simulink library "INT_ACCmpr_DD"  (R2016b)
settings: Solver=VariableStepAuto  StartTime=0.0  StopTime=10.0  RelTol=1e-3
settings Model: Creator=liutao  LastModifiedBy=liutao

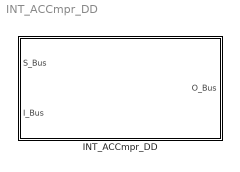
== system INT_ACCmpr_DD ==
  INT_ACCmpr_DD : Subsystem

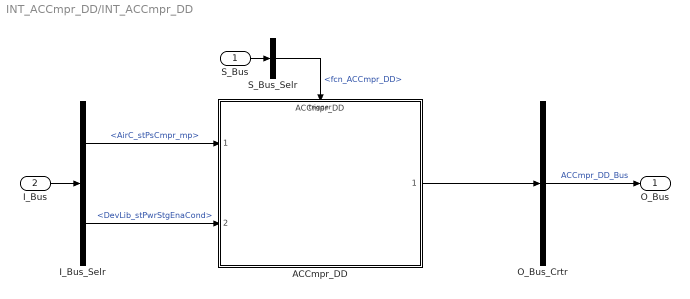
== system INT_ACCmpr_DD/INT_ACCmpr_DD ==
  S_Bus : Inport
  I_Bus : Inport  Port=2
  ACCmpr_DD : ModelReference  ModelNameDialog=ACCmpr_DD  SimulationMode=Normal  ModelReferenceVersion=1.14  TriggerPortName=function  TriggerPortTriggerType=function-call  TriggerPortStatesWhenEnabling=held
  I_Bus_Selr : BusSelector  OutputSignals=AirC_stPsCmpr_mp,DevLib_stPwrStgEnaCond
  O_Bus_Crtr : BusCreator  Inputs=1
  S_Bus_Selr : BusSelector  OutputSignals=fcn_ACCmpr_DD
  O_Bus : Outport
  wires:
  S_Bus_Selr/1 -> ACCmpr_DD/Trigger  "<fcn_ACCmpr_DD>"
  S_Bus/1 -> S_Bus_Selr/1
  I_Bus/1 -> I_Bus_Selr/1
  I_Bus_Selr/1 -> ACCmpr_DD/1  "<AirC_stPsCmpr_mp>"
  I_Bus_Selr/2 -> ACCmpr_DD/2  "<DevLib_stPwrStgEnaCond>"
  O_Bus_Crtr/1 -> O_Bus/1  "ACCmpr_DD_Bus"
  ACCmpr_DD/1 -> O_Bus_Crtr/1
